simulink model "week23"  (R2020a)
settings: Solver=ode45  StartTime=0.0  StopTime=120  RelTol=1e-3
values from neighbouring files (symbols this model uses):
  m = 1000    [ccm.mat]
settings Model: Creator=Admin  LastModifiedBy=Admin

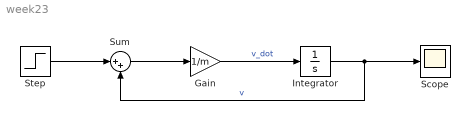
== system week23 ==
  Gain : Gain  Gain=1/m
  Integrator : Integrator
  Scope : Scope
  Step : Step  Time=0  After=u  SampleTime=0
  Sum : Sum  Inputs=|++
  wires:
  Gain/1 -> Integrator/1  "v_dot"
  Sum/1 -> Gain/1
  Integrator/1 -> Sum/2, Scope/1  "v"
  Step/1 -> Sum/1
